simulink model "FinalProject"  (R2022b)
settings: Solver=ode1be  StartTime=0.0  StopTime=10  FixedStep=0.001  RelTol=1e-3
libraries: simulink x1
settings Model: Creator=Ilya_Andriyanov  LastModifiedBy=Ilya_Andriyanov
settings SolverCC: ZeroCrossAlgorithm=Adaptive  SolverResetMethod=Robust

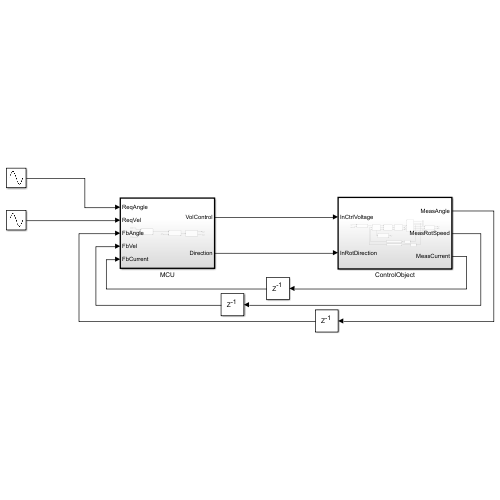
[thumbnail: Simulink's stored preview of the top-level diagram]
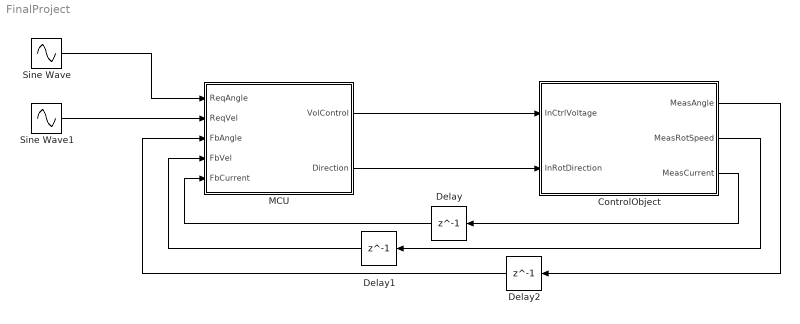
== system FinalProject ==
  ControlObject : Subsystem  TreatAsAtomicUnit=on
  Delay : Delay  DelayLength=1
  Delay1 : Delay  DelayLength=1
  Delay2 : Delay  DelayLength=1
  MCU : Subsystem  TreatAsAtomicUnit=on
  Sine Wave : Sin  Amplitude=0.5  Frequency=10  SampleTime=0
  Sine Wave1 : Sin  Amplitude=0.5  Frequency=10  Phase=pi/2  SampleTime=0
  wires:
  Sine Wave/1 -> MCU/1(ReqAngle)
  ControlObject/3(MeasCurrent) -> Delay/1
  ControlObject/2(MeasRotSpeed) -> Delay1/1
  ControlObject/1(MeasAngle) -> Delay2/1
  Sine Wave1/1 -> MCU/2(ReqVel)
  MCU/2(Direction) -> ControlObject/2(InRotDirection)
  MCU/1(VolControl) -> ControlObject/1(InCtrlVoltage)
  Delay/1 -> MCU/5(FbCurrent)
  Delay1/1 -> MCU/4(FbVel)
  Delay2/1 -> MCU/3(FbAngle)

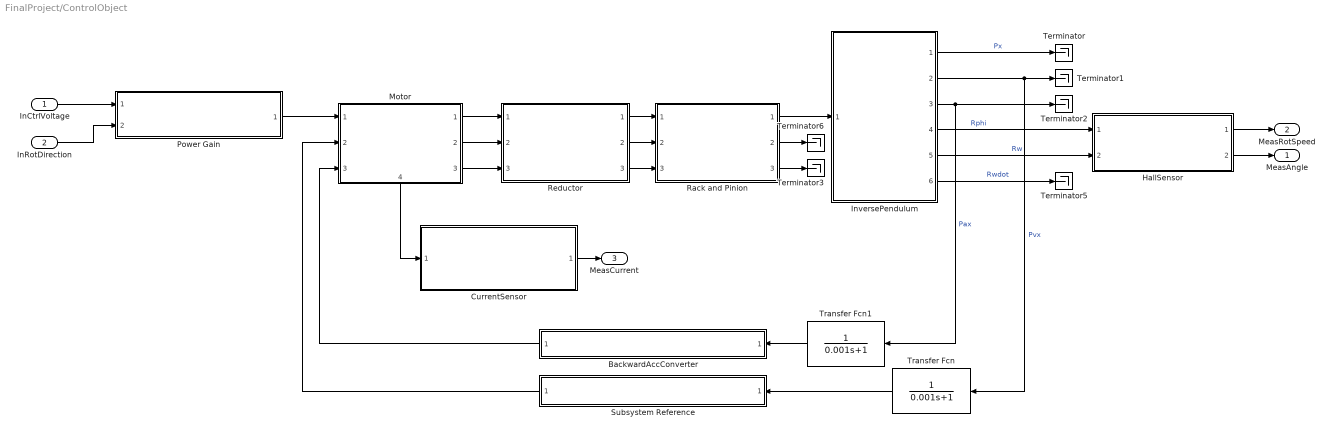
== system FinalProject/ControlObject ==
  InCtrlVoltage : Inport
  InRotDirection : Inport  Port=2
  BackwardAccConverter : Subsystem  ReferencedSubsystem=BackwardConverter
  CurrentSensor : Subsystem  ReferencedSubsystem=CurrentSensor
  HallSensor : Subsystem  ReferencedSubsystem=HallSensor
  InversePendulum : Subsystem  ReferencedSubsystem=InversePendulum
  Motor : Subsystem  ReferencedSubsystem=DCMotor
      settings: PortSchema="{\"entries\":[{\"content\":{\"sides\":[{\"content\":{\"connectorIds\":[\"In1\",\"In2\",\"In3\"]},\"type\":\"ConnectorPlacement.EquallySpacedRectSide\",\"uuid\":\"cf1f6aad-091f-4111-96d2-0ff15b1f9161\"},{\"content\":{\"connectorIds\":[\"Out1\",\"Out2\",\"Out3\"],\"side\":\"RIGHT\"},\"type\":\"ConnectorPlacement.EquallySpacedRectSide\",\"uuid\":\"4922c734-6a98-471f-9783-d3bdbedc5471\"},{\"content\":{\"connectorIds\":[],\"side\":\"TOP\"},\"type\":\"ConnectorPlacement.EquallySpacedRectSide\",\"uuid\":\"3fe4576c-eff2-4c07-9e6e-2ac91bc88fc0\"},{\"content\":{\"connectorIds\":[\"Out4\"],\"side\":\"BOTTOM\"},\"type\":\"ConnectorPlacement.EquallySpacedRectSide\",\"uuid\":\"5386b3f7-eb9a-4d61-b7f7-90b2df797b5b\"}]},\"type\":\"ConnectorPlacement.EquallySpacedConnector\",\"uuid\":\"65c52474-0e26-40fa-9f38-b3d27a4921a2\"}],\"packageUris\":[\"http://schema.mathworks.com/mf0/Connector/R2020b\"],\"version\":\"1.0\"}"
  Power Gain : Subsystem  ReferencedSubsystem=PowerGain
  Rack and Pinion : Subsystem  ReferencedSubsystem=RackAndPinion
  Reductor : Subsystem  ReferencedSubsystem=Reductor
  Subsystem Reference : Subsystem  ReferencedSubsystem=BackwardConverter
  Terminator{,1..3,5..6} (6 alike) : Terminator
  Transfer Fcn : TransferFcn  Denominator=[0.001 1]
  Transfer Fcn1 : TransferFcn  Denominator=[0.001 1]
  MeasAngle : Outport
  MeasRotSpeed : Outport  Port=2
  MeasCurrent : Outport  Port=3
  wires:
  InversePendulum/4 -> HallSensor/1  "Rphi"
  Motor/1 -> Reductor/1
  Motor/2 -> Reductor/2
  Reductor/2 -> Rack and Pinion/2
  Reductor/1 -> Rack and Pinion/1
  Rack and Pinion/2 -> Terminator6/1
  InversePendulum/3 -> Terminator2/1, Transfer Fcn1/1  "Pax"
  InversePendulum/6 -> Terminator5/1  "Rwdot"
  InversePendulum/2 -> Terminator1/1, Transfer Fcn/1  "Pvx"
  InversePendulum/1 -> Terminator/1  "Px"
  InversePendulum/5 -> HallSensor/2  "Rw"
  Rack and Pinion/1 -> InversePendulum/1
  HallSensor/1 -> MeasRotSpeed/1
  HallSensor/2 -> MeasAngle/1
  Motor/4 -> CurrentSensor/1
  CurrentSensor/1 -> MeasCurrent/1
  Power Gain/1 -> Motor/1
  InCtrlVoltage/1 -> Power Gain/1
  InRotDirection/1 -> Power Gain/2
  Motor/3 -> Reductor/3
  Reductor/3 -> Rack and Pinion/3
  Rack and Pinion/3 -> Terminator3/1
  BackwardAccConverter/1 -> Motor/3
  Subsystem Reference/1 -> Motor/2
  Transfer Fcn/1 -> Subsystem Reference/1
  Transfer Fcn1/1 -> BackwardAccConverter/1

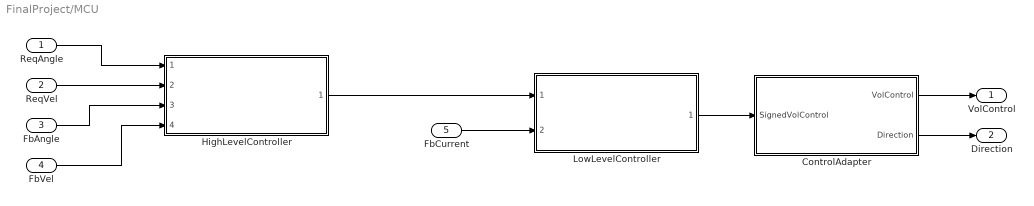
== system FinalProject/MCU ==
  ReqAngle : Inport
  ReqVel : Inport  Port=2
  FbAngle : Inport  Port=3
  FbVel : Inport  Port=4
  FbCurrent : Inport  Port=5
  ControlAdapter : Subsystem
  HighLevelController : Subsystem  ReferencedSubsystem=HighLevelController
  LowLevelController : Subsystem  ReferencedSubsystem=LowLevelController
  VolControl : Outport
  Direction : Outport  Port=2
  wires:
  FbCurrent/1 -> LowLevelController/2
  ReqAngle/1 -> HighLevelController/1
  HighLevelController/1 -> LowLevelController/1
  FbVel/1 -> HighLevelController/4
  FbAngle/1 -> HighLevelController/3
  ControlAdapter/1(VolControl) -> VolControl/1
  ControlAdapter/2(Direction) -> Direction/1
  LowLevelController/1 -> ControlAdapter/1(SignedVolControl)
  ReqVel/1 -> HighLevelController/2

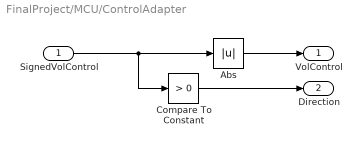
== system FinalProject/MCU/ControlAdapter ==
  SignedVolControl : Inport
  Abs : Abs  SaturateOnIntegerOverflow=off
  Compare To Constant : simulink/Logic and Bit Operations/Compare To Constant  relop=>  const=0  OutDataTypeStr=boolean
  VolControl : Outport
  Direction : Outport  Port=2
  wires:
  Compare To Constant/1 -> Direction/1
  SignedVolControl/1 -> Abs/1, Compare To Constant/1
  Abs/1 -> VolControl/1
